simulink model "assignment2_group39_v10_final"  (R2022b)
settings: Solver=FixedStepAuto  StartTime=0.0  StopTime=30  FixedStep=0.001  RelTol=1e-3  EnableMultiTasking=on
undefined symbols (not defined in the file): A0, A1, D0, D1, D10, D11, D12, D13, D2, D3, D4, D5, D6, D7, D8, D9, PTA0, PTA1, PTA2, PTB2, PTB23, PTB3, PTB9, PTC16, PTC17, PTC2, PTC3, PTC4, PTD0, PTD1, PTD2, PTD3
libraries: frdmk64flib x24, etargetslib x16, dspstat3 x1
settings Model: ExtModeTrigDuration=5  Creator=andre  LastModifiedBy=Jack Mann
settings SolverCC: AlgebraicLoopSolver=TrustRegion
settings OptimizationCC: EnhancedBackFolding=on  PassReuseOutputArgsAs=Individual arguments  ZeroExternalMemoryAtStartup=off  ZeroInternalMemoryAtStartup=off  MaxStackSize=64  OptimizeBlockOrder=speed  DifferentSizesBufferReuse=on  OptimizationCustomize=off  EfficientTunableParamExpr=on
settings DebuggingCC: ParameterTunabilityLossMsg=error  UnconnectedInputMsg=warning  UnconnectedOutputMsg=warning  UnconnectedLineMsg=warning
settings HardwareCC: ProdBitPerPointer=32  ProdBitPerSizeT=32  ProdBitPerPtrDiffT=32  ProdLargestAtomicInteger=Long  ProdLargestAtomicFloat=Double  ProdWordSize=32  ProdHWDeviceType=ARM Compatible->ARM Cortex
settings ModelReferenceCC: EnableRefExpFcnMdlSchedulingChecks=on
settings SFSimCC: MATLABDynamicMemAlloc=off
settings RTWCC: Description=Embedded Coder  SystemTargetFile=ert.tlc  HardwareBoard=NXP FRDM-K64F  TLCOptions="-aInlineSetEventsForThisBaseRateFcn=TLC_FALSE -aSuppressMultiTaskScheduler=TLC_FALSE  -aRateBasedStepFcn=0"  TemplateMakefile=ert_default_tmf  Toolchain=GNU Tools for ARM Embedded Processors
settings CodeAppCC: ForceParamTrailComments=on  IgnoreCustomStorageClasses=off  OperatorAnnotations=on  SimulinkDataObjDesc=on  SFDataObjDesc=on  InsertBlockDesc=on

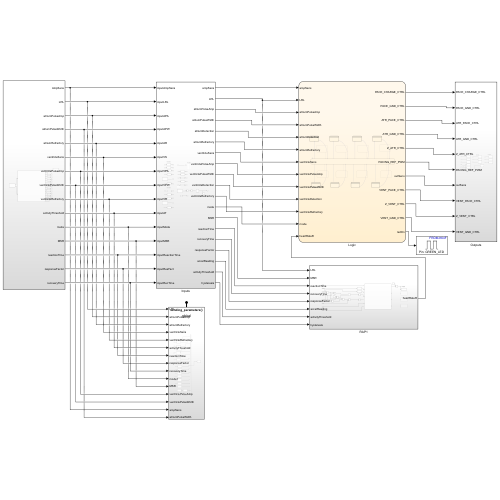
[thumbnail: Simulink's stored preview of the top-level diagram]
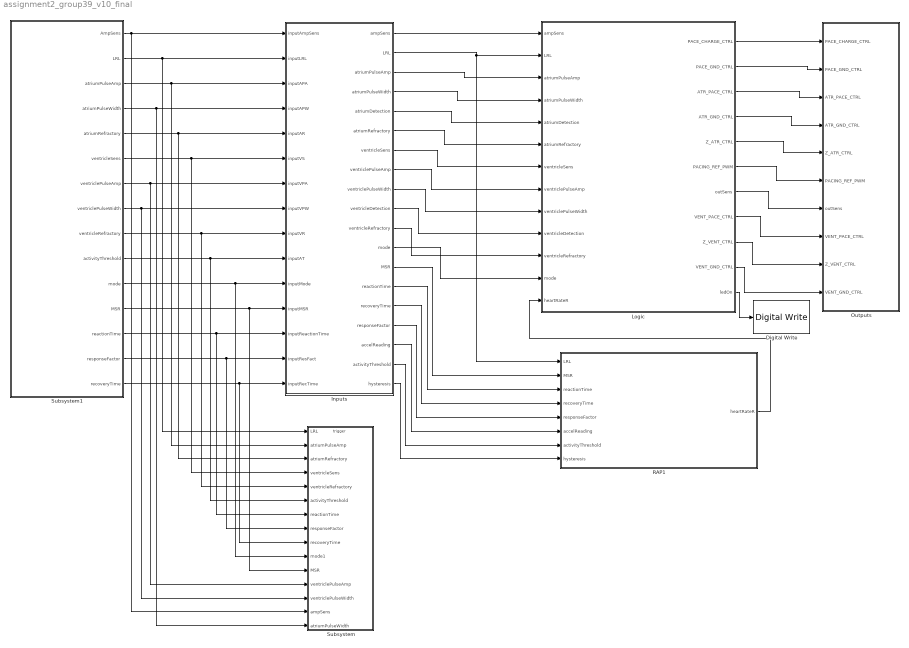
== system assignment2_group39_v10_final ==
  Digital Write : frdmk64flib/Digital Write  Whichpin=GREEN_LED
  Inputs : Subsystem
  Logic : Stateflow chart  TreatAsAtomicUnit=on
  Outputs : Subsystem
  RAP1 : Subsystem
  Subsystem : Subsystem
  Subsystem1 : Subsystem
  wires:
  Inputs/1(ampSens) -> Logic/1(ampSens)
  Inputs/2(LRL) -> RAP1/1(LRL), Logic/2(LRL)
  Inputs/3(atriumPulseAmp) -> Logic/3(atriumPulseAmp)
  Inputs/4(atriumPulseWidth) -> Logic/4(atriumPulseWidth)
  Inputs/5(atriumDetection) -> Logic/5(atriumDetection)
  Inputs/6(atriumRefractory) -> Logic/6(atriumRefractory)
  Logic/1(PACE_CHARGE_CTRL) -> Outputs/1(PACE_CHARGE_CTRL)
  Logic/2(PACE_GND_CTRL) -> Outputs/2(PACE_GND_CTRL)
  Logic/3(ATR_PACE_CTRL) -> Outputs/3(ATR_PACE_CTRL)
  Logic/4(ATR_GND_CTRL) -> Outputs/4(ATR_GND_CTRL)
  Logic/5(Z_ATR_CTRL) -> Outputs/5(Z_ATR_CTRL)
  Logic/6(PACING_REF_PWM) -> Outputs/6(PACING_REF_PWM)
  Logic/7(outSens) -> Outputs/7(outSens)
  Inputs/7(ventricleSens) -> Logic/7(ventricleSens)
  Inputs/8(ventriclePulseAmp) -> Logic/8(ventriclePulseAmp)
  Inputs/9(ventriclePulseWidth) -> Logic/9(ventriclePulseWidth)
  Inputs/10(ventricleDetection) -> Logic/10(ventricleDetection)
  Inputs/11(ventricleRefractory) -> Logic/11(ventricleRefractory)
  Logic/8(VENT_PACE_CTRL) -> Outputs/8(VENT_PACE_CTRL)
  Logic/9(Z_VENT_CTRL) -> Outputs/9(Z_VENT_CTRL)
  Logic/10(VENT_GND_CTRL) -> Outputs/10(VENT_GND_CTRL)
  Inputs/12(mode) -> Logic/12(mode)
  Inputs/13(MSR) -> RAP1/2(MSR)
  Inputs/16(responseFactor) -> RAP1/5(responseFactor)
  Inputs/14(reactionTime) -> RAP1/3(reactionTime)
  Inputs/15(recoveryTime) -> RAP1/4(recoveryTime)
  Inputs/18(activityThreshold) -> RAP1/7(activityThreshold)
  Inputs/17(accelReading) -> RAP1/6(accelReading)
  RAP1/1(heartRateR) -> Logic/13(heartRateR)
  Subsystem1/1(AmpSens) -> Subsystem/14(ampSens), Inputs/1(inputAmpSens)
  Subsystem1/3(atriumPulseAmp) -> Subsystem/2(atriumPulseAmp), Inputs/3(inputAPA)
  Subsystem1/4(atriumPulseWidth) -> Subsystem/15(atriumPulseWidth), Inputs/4(inputAPW)
  Subsystem1/6(ventricleSens) -> Subsystem/4(ventricleSens), Inputs/6(inputVS)
  Subsystem1/7(ventriclePulseAmp) -> Subsystem/12(ventriclePulseAmp), Inputs/7(inputVPA)
  Subsystem1/8(ventriclePulseWidth) -> Subsystem/13(ventriclePulseWidth), Inputs/8(inputVPW)
  Subsystem1/9(ventricleRefractory) -> Subsystem/5(ventricleRefractory), Inputs/9(inputVR)
  Subsystem1/14(responseFactor) -> Subsystem/8(responseFactor), Inputs/14(inputResFact)
  Subsystem1/15(recoveryTime) -> Subsystem/9(recoveryTime), Inputs/15(inputRecTime)
  Subsystem1/10(activityThreshold) -> Subsystem/6(activityThreshold), Inputs/10(inputAT)
  Subsystem1/11(mode) -> Subsystem/10(mode1), Inputs/11(inputMode)
  Subsystem1/12(MSR) -> Subsystem/11(MSR), Inputs/12(inputMSR)
  Subsystem1/13(reactionTime) -> Subsystem/7(reactionTime), Inputs/13(inputReactionTime)
  Inputs/19(hysteresis) -> RAP1/8(hysteresis)
  Subsystem1/2(LRL) -> Subsystem/1(LRL), Inputs/2(inputLRL)
  Subsystem1/5(atriumRefractory) -> Subsystem/3(atriumRefractory), Inputs/5(inputAR)
  Logic/11(ledOn) -> Digital Write/1

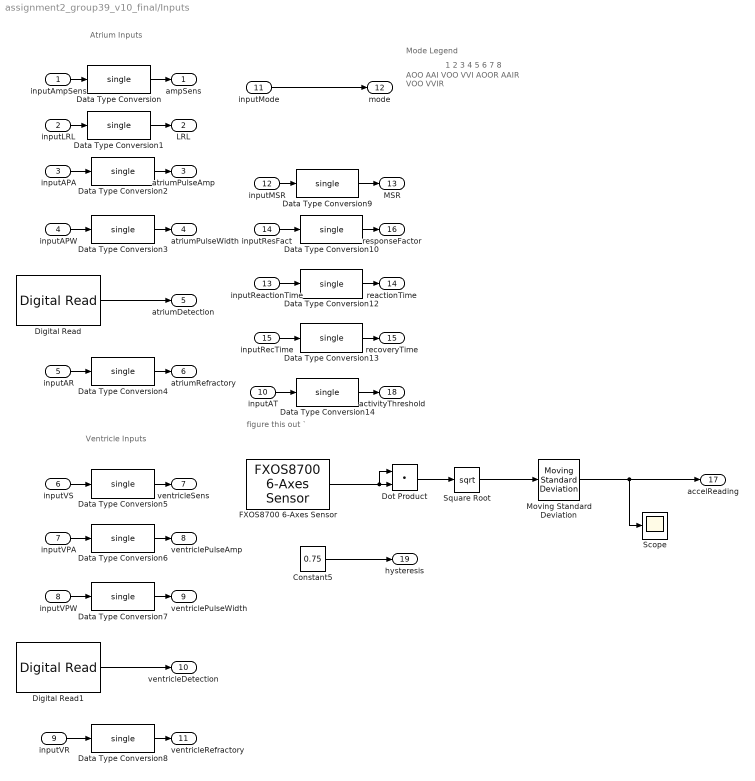
== system assignment2_group39_v10_final/Inputs ==
  note: 1
      | 2
      | 3
      | 4
      | 5
      | 6
      | 7
      | 8
  note: figure this out
      | `
  note: Mode Legend
  note: AOO
      | AAI
      | VOO
      | VVI
      | AOOR
      | AAIR
      | VOO
      | VVIR
  note: Ventricle Inputs
  note: Atrium Inputs
  inputAmpSens : Inport
  inputLRL : Inport  Port=2
  inputAPA : Inport  Port=3
  inputAPW : Inport  Port=4
  inputAR : Inport  Port=5
  inputVS : Inport  Port=6
  inputVPA : Inport  Port=7
  inputVPW : Inport  Port=8
  inputVR : Inport  Port=9
  inputAT : Inport  Port=10
  inputMode : Inport  Port=11
  inputMSR : Inport  Port=12
  inputReactionTime : Inport  Port=13
  inputResFact : Inport  Port=14
  inputRecTime : Inport  Port=15
  Constant5 : Constant  Value=0.75
  Data Type Conversion{,1..10,12..14} (14 alike) : DataTypeConversion  OutDataTypeStr=single  SaturateOnIntegerOverflow=off  RndMeth=Floor
  Digital Read : frdmk64flib/Digital Read  Whichpin=PTC16 (D0)  SampleTime=-1
  Digital Read1 : frdmk64flib/Digital Read  Whichpin=PTC17 (D1)  SampleTime=-1
  Dot Product : DotProduct  OutDataTypeStr=Inherit: Inherit via internal rule
  FXOS8700 6-Axes Sensor : frdmk64flib/FXOS8700 6-Axes Sensor  Activesensor=Accelerometer only  ODR=800Hz  HybridODR=400Hz  Accelfullrange=-4g to +4g  SampleTime=-1
  Moving Standard Deviation : dspstat3/Moving Standard Deviation  Method=Sliding window  ForgettingFactorPort=off  SpecifyWindowLength=on  WindowLength=4  OverlapLength=3  AllowArbitraryInputLength=off  ForgettingFactor=0.9  SimulateUsing=Code generation
  Scope : Scope
  Square Root : Sqrt
  ampSens : Outport  OutDataTypeStr=single
  LRL : Outport  Port=2  OutDataTypeStr=single
  atriumPulseAmp : Outport  Port=3  OutDataTypeStr=single
  atriumPulseWidth : Outport  Port=4  OutDataTypeStr=single
  atriumDetection : Outport  Port=5  OutDataTypeStr=boolean
  atriumRefractory : Outport  Port=6  OutDataTypeStr=single
  ventricleSens : Outport  Port=7  OutDataTypeStr=single
  ventriclePulseAmp : Outport  Port=8  OutDataTypeStr=single
  ventriclePulseWidth : Outport  Port=9  OutDataTypeStr=single
  ventricleDetection : Outport  Port=10  OutDataTypeStr=boolean
  ventricleRefractory : Outport  Port=11  OutDataTypeStr=single
  mode : Outport  Port=12  OutDataTypeStr=uint8
  MSR : Outport  Port=13
  reactionTime : Outport  Port=14
  recoveryTime : Outport  Port=15
  responseFactor : Outport  Port=16
  accelReading : Outport  Port=17
  activityThreshold : Outport  Port=18
  hysteresis : Outport  Port=19
  wires:
  inputAmpSens/1 -> Data Type Conversion/1
  inputAPW/1 -> Data Type Conversion3/1
  inputAR/1 -> Data Type Conversion4/1
  inputAPA/1 -> Data Type Conversion2/1
  inputLRL/1 -> Data Type Conversion1/1
  Digital Read/1 -> atriumDetection/1
  Digital Read1/1 -> ventricleDetection/1
  inputVPW/1 -> Data Type Conversion7/1
  inputVPA/1 -> Data Type Conversion6/1
  inputVR/1 -> Data Type Conversion8/1
  inputVS/1 -> Data Type Conversion5/1
  inputMSR/1 -> Data Type Conversion9/1
  inputResFact/1 -> Data Type Conversion10/1
  inputReactionTime/1 -> Data Type Conversion12/1
  inputRecTime/1 -> Data Type Conversion13/1
  inputAT/1 -> Data Type Conversion14/1
  FXOS8700 6-Axes Sensor/1 -> Dot Product/1, Dot Product/2
  Dot Product/1 -> Square Root/1
  Square Root/1 -> Moving Standard Deviation/1
  Data Type Conversion/1 -> ampSens/1
  Data Type Conversion1/1 -> LRL/1
  Data Type Conversion2/1 -> atriumPulseAmp/1
  Data Type Conversion3/1 -> atriumPulseWidth/1
  Data Type Conversion4/1 -> atriumRefractory/1
  Data Type Conversion5/1 -> ventricleSens/1
  Data Type Conversion6/1 -> ventriclePulseAmp/1
  Data Type Conversion7/1 -> ventriclePulseWidth/1
  Data Type Conversion8/1 -> ventricleRefractory/1
  Data Type Conversion9/1 -> MSR/1
  Data Type Conversion10/1 -> responseFactor/1
  inputMode/1 -> mode/1
  Data Type Conversion12/1 -> reactionTime/1
  Data Type Conversion13/1 -> recoveryTime/1
  Data Type Conversion14/1 -> activityThreshold/1
  Constant5/1 -> hysteresis/1
  Moving Standard Deviation/1 -> Scope/1, accelReading/1

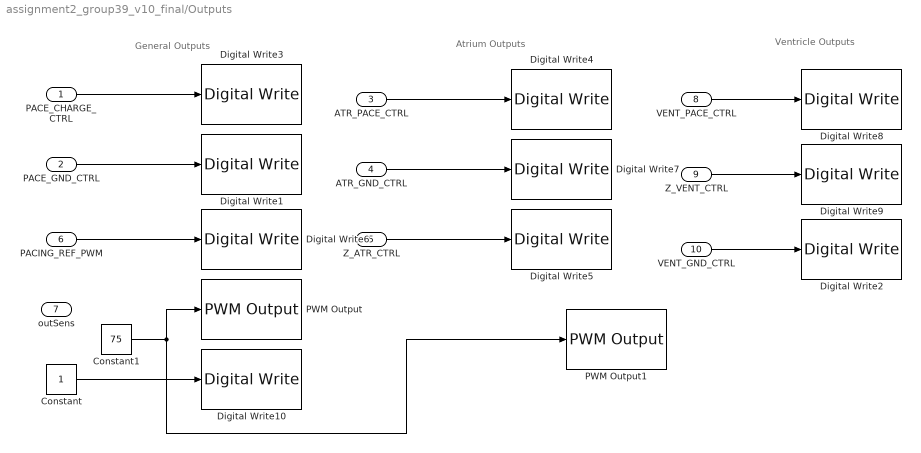
== system assignment2_group39_v10_final/Outputs ==
  note: Ventricle Outputs
  note: Atrium Outputs
  note: General Outputs
  PACE_CHARGE_CTRL : Inport  OutDataTypeStr=boolean
  PACE_GND_CTRL : Inport  Port=2  OutDataTypeStr=boolean
  ATR_PACE_CTRL : Inport  Port=3  OutDataTypeStr=boolean
  ATR_GND_CTRL : Inport  Port=4  OutDataTypeStr=boolean
  Z_ATR_CTRL : Inport  Port=5  OutDataTypeStr=boolean
  PACING_REF_PWM : Inport  Port=6  OutDataTypeStr=single
  outSens : Inport  Port=7  OutDataTypeStr=single
  VENT_PACE_CTRL : Inport  Port=8  OutDataTypeStr=boolean
  Z_VENT_CTRL : Inport  Port=9  OutDataTypeStr=boolean
  VENT_GND_CTRL : Inport  Port=10  OutDataTypeStr=boolean
  Constant : Constant  OutDataTypeStr=single
  Constant1 : Constant  Value=75
  Digital Write1 : frdmk64flib/Digital Write  Whichpin=PTD0 (D10)
  Digital Write10 : frdmk64flib/Digital Write  Whichpin=PTD1 (D13)
  Digital Write2 : frdmk64flib/Digital Write  Whichpin=PTD3 (D12)
  Digital Write3 : frdmk64flib/Digital Write  Whichpin=PTB9 (D2)
  Digital Write4 : frdmk64flib/Digital Write  Whichpin=PTA0 (D8)
  Digital Write5 : frdmk64flib/Digital Write  Whichpin=PTB23 (D4)
  Digital Write6 : frdmk64flib/Digital Write  Whichpin=PTA2 (D5)
  Digital Write7 : frdmk64flib/Digital Write  Whichpin=PTD2 (D11)
  Digital Write8 : frdmk64flib/Digital Write  Whichpin=PTC4 (D9)
  Digital Write9 : frdmk64flib/Digital Write  Whichpin=PTC3 (D7)
  PWM Output : frdmk64flib/PWM Output  Whichpin=PTC2 (D6)  InitialFrequency=2000  InitialDutyCycle=0
  PWM Output1 : frdmk64flib/PWM Output  Whichpin=PTA1 (D3)  InitialFrequency=2000  InitialDutyCycle=0
  wires:
  PACING_REF_PWM/1 -> Digital Write6/1
  ATR_PACE_CTRL/1 -> Digital Write4/1
  PACE_CHARGE_CTRL/1 -> Digital Write3/1
  Z_ATR_CTRL/1 -> Digital Write5/1
  ATR_GND_CTRL/1 -> Digital Write7/1
  Constant/1 -> Digital Write10/1
  PACE_GND_CTRL/1 -> Digital Write1/1
  Z_VENT_CTRL/1 -> Digital Write9/1
  VENT_GND_CTRL/1 -> Digital Write2/1
  VENT_PACE_CTRL/1 -> Digital Write8/1
  Constant1/1 -> PWM Output1/1, PWM Output/1

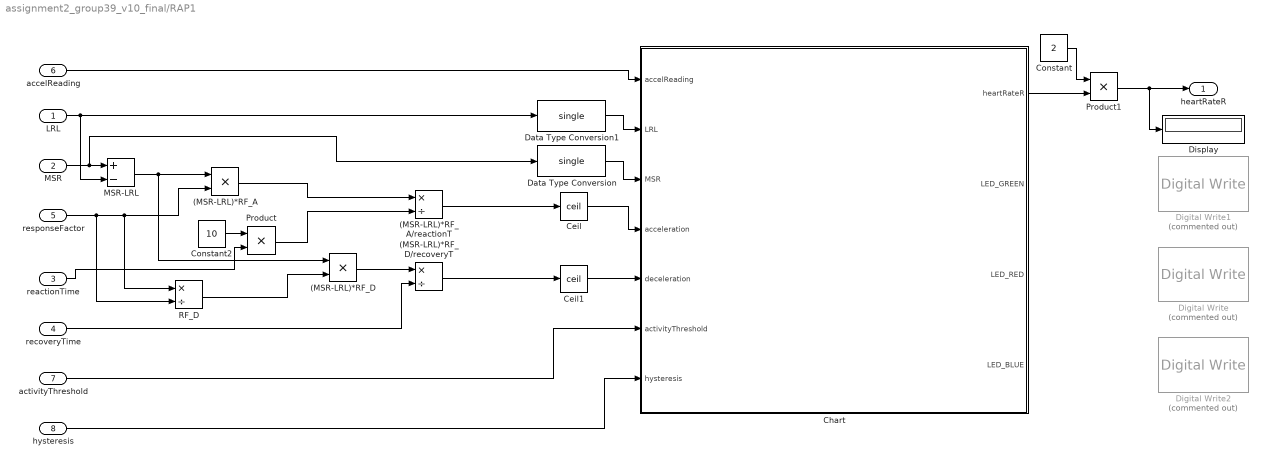
== system assignment2_group39_v10_final/RAP1 ==
  LRL : Inport
  MSR : Inport  Port=2
  reactionTime : Inport  Port=3
  recoveryTime : Inport  Port=4
  responseFactor : Inport  Port=5
  accelReading : Inport  Port=6
  activityThreshold : Inport  Port=7
  hysteresis : Inport  Port=8
  (MSR-LRL)*RF_A : Product
  (MSR-LRL)*RF_A/reactionT : Product  Inputs=*/
  (MSR-LRL)*RF_D : Product
  (MSR-LRL)*RF_D/recoveryT : Product  Inputs=*/
  Ceil : Rounding  Operator=ceil
  Ceil1 : Rounding  Operator=ceil
  Chart : Stateflow chart  TreatAsAtomicUnit=on
      settings: PortSchema="{\"entries\":[{\"content\":{\"sides\":[{\"content\":{\"connectorIds\":[\"In4\",\"In1\",\"In6\",\"In2\",\"In5\",\"In3\",\"In7\"]},\"type\":\"ConnectorPlacement.EquallySpacedRectSide\",\"uuid\":\"e727a920-989a-48c2-8c82-674329886a5f\"},{\"content\":{\"connectorIds\":[\"Out1\",\"Out3\",\"Out2\",\"Out4\"],\"side\":\"RIGHT\"},\"type\":\"ConnectorPlacement.EquallySpacedRectSide\",\"uuid\":\"1ee40f3e-9295-4daa-a641-24f0111d1364\"},{\"content\":{\"side\":\"TOP\"},\"type\":\"ConnectorPlacement.EquallySpacedRectSide\",\"uuid\":\"e3e534e8-f7ca-4b9e-96df-b8a39382b9c4\"}]},\"type\":\"ConnectorPlacement.EquallySpacedConnector\",\"uuid\":\"172b69cd-74db-4b29-a177-e1757147670c\"}],\"packageUris\":[\"http://schema.mathworks.com/mf0/Connector/R2020b\"],\"version\":\"1.0\"}"
  Constant : Constant  Value=2  OutDataTypeStr=single
  Constant2 : Constant  Value=10
  Data Type Conversion : DataTypeConversion  OutDataTypeStr=single  SaturateOnIntegerOverflow=off  RndMeth=Floor
  Data Type Conversion1 : DataTypeConversion  OutDataTypeStr=single  SaturateOnIntegerOverflow=off  RndMeth=Floor
  Digital Write : frdmk64flib/Digital Write  Commented=on  Whichpin=RED_LED
  Digital Write1 : frdmk64flib/Digital Write  Commented=on  Whichpin=GREEN_LED
  Digital Write2 : frdmk64flib/Digital Write  Commented=on  Whichpin=BLUE_LED
  Display : Display
  MSR-LRL : Sum  Inputs=+-
  Product : Product
  Product1 : Product
  RF_D : Product  Inputs=*/
  heartRateR : Outport
  wires:
  LRL/1 -> MSR-LRL/2, Data Type Conversion1/1
  accelReading/1 -> Chart/4(accelReading)
  MSR/1 -> Data Type Conversion/1, MSR-LRL/1
  MSR-LRL/1 -> (MSR-LRL)*RF_D/1, (MSR-LRL)*RF_A/1
  responseFactor/1 -> RF_D/2, RF_D/1, (MSR-LRL)*RF_A/2
  (MSR-LRL)*RF_A/1 -> (MSR-LRL)*RF_A/reactionT/1
  recoveryTime/1 -> (MSR-LRL)*RF_D/recoveryT/2
  Ceil/1 -> Chart/2(acceleration)
  (MSR-LRL)*RF_A/reactionT/1 -> Ceil/1
  (MSR-LRL)*RF_D/1 -> (MSR-LRL)*RF_D/recoveryT/1
  (MSR-LRL)*RF_D/recoveryT/1 -> Ceil1/1
  activityThreshold/1 -> Chart/3(activityThreshold)
  hysteresis/1 -> Chart/7(hysteresis)
  Data Type Conversion/1 -> Chart/6(MSR)
  Data Type Conversion1/1 -> Chart/1(LRL)
  Product1/1 -> heartRateR/1, Display/1
  Ceil1/1 -> Chart/5(deceleration)
  Product/1 -> (MSR-LRL)*RF_A/reactionT/2
  Constant2/1 -> Product/1
  reactionTime/1 -> Product/2
  RF_D/1 -> (MSR-LRL)*RF_D/2
  Chart/1(heartRateR) -> Product1/2
  Constant/1 -> Product1/1

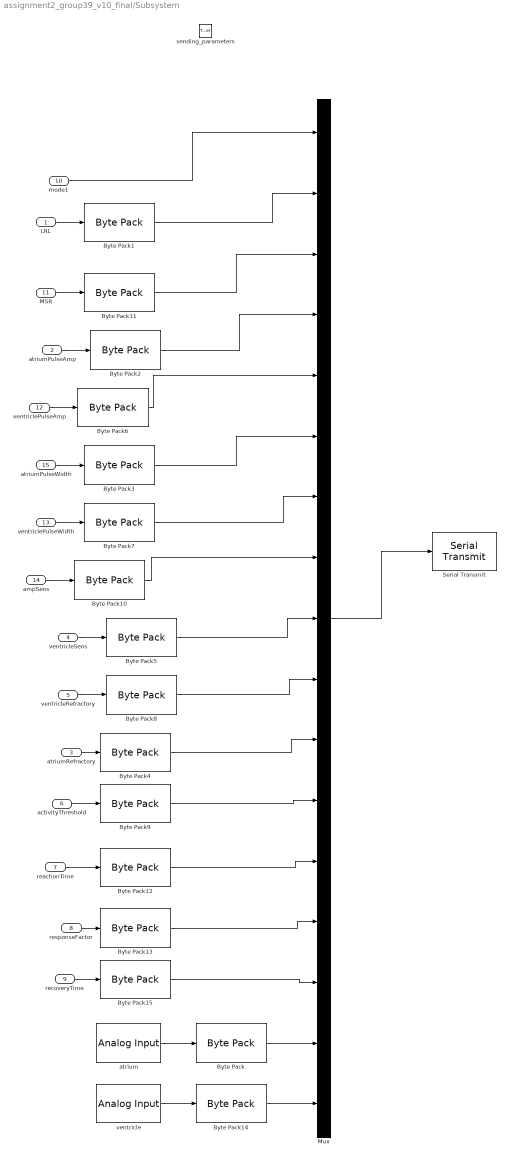
== system assignment2_group39_v10_final/Subsystem ==
  LRL : Inport  OutDataTypeStr=double
  atriumPulseAmp : Inport  Port=2  OutDataTypeStr=double
  atriumRefractory : Inport  Port=3  OutDataTypeStr=double
  ventricleSens : Inport  Port=4  OutDataTypeStr=double
  ventricleRefractory : Inport  Port=5  OutDataTypeStr=double
  activityThreshold : Inport  Port=6  OutDataTypeStr=double
  reactionTime : Inport  Port=7  OutDataTypeStr=double
  responseFactor : Inport  Port=8  OutDataTypeStr=double
  recoveryTime : Inport  Port=9  OutDataTypeStr=double
  mode1 : Inport  Port=10  OutDataTypeStr=uint8
  MSR : Inport  Port=11  OutDataTypeStr=double
  ventriclePulseAmp : Inport  Port=12  OutDataTypeStr=double
  ventriclePulseWidth : Inport  Port=13  OutDataTypeStr=double
  ampSens : Inport  Port=14  OutDataTypeStr=double
  atriumPulseWidth : Inport  Port=15  OutDataTypeStr=double
  sending_parameters : TriggerPort  TriggerType=function-call  IsSimulinkFunction=on  FunctionName=sending_parameters  VariantControl=Variant
  Byte Pack{,1..15} (16 alike) : etargetslib/Byte Pack  datatypes={'double'}  byteAlign=1
  Mux : Mux  Inputs=17
  Serial Transmit : frdmk64flib/Serial Transmit  SCIModule=0  Baudrate=uint32(9600)  Parity=None  StopBits=1  HardwareFlowControl=None  ByteOrder=LittleEndian  BlockingMode=on  OutputStatus=off
  atrium : frdmk64flib/Analog Input  Whichpin=PTB2 (A0)  SampleTime=-1
  ventricle : frdmk64flib/Analog Input  Whichpin=PTB3 (A1)  SampleTime=-1
  wires:
  LRL/1 -> Byte Pack1/1
  atriumPulseAmp/1 -> Byte Pack2/1
  atriumRefractory/1 -> Byte Pack4/1
  ventricleSens/1 -> Byte Pack5/1
  ventricleRefractory/1 -> Byte Pack8/1
  activityThreshold/1 -> Byte Pack9/1
  reactionTime/1 -> Byte Pack12/1
  responseFactor/1 -> Byte Pack13/1
  recoveryTime/1 -> Byte Pack15/1
  Mux/1 -> Serial Transmit/1
  MSR/1 -> Byte Pack11/1
  Byte Pack11/1 -> Mux/3
  ventriclePulseAmp/1 -> Byte Pack6/1
  ventriclePulseWidth/1 -> Byte Pack7/1
  ampSens/1 -> Byte Pack10/1
  atriumPulseWidth/1 -> Byte Pack3/1
  Byte Pack15/1 -> Mux/15
  Byte Pack13/1 -> Mux/14
  Byte Pack12/1 -> Mux/13
  Byte Pack9/1 -> Mux/12
  Byte Pack4/1 -> Mux/11
  Byte Pack8/1 -> Mux/10
  Byte Pack5/1 -> Mux/9
  Byte Pack10/1 -> Mux/8
  Byte Pack7/1 -> Mux/7
  Byte Pack3/1 -> Mux/6
  Byte Pack6/1 -> Mux/5
  Byte Pack2/1 -> Mux/4
  Byte Pack1/1 -> Mux/2
  mode1/1 -> Mux/1
  atrium/1 -> Byte Pack/1
  ventricle/1 -> Byte Pack14/1
  Byte Pack/1 -> Mux/16
  Byte Pack14/1 -> Mux/17

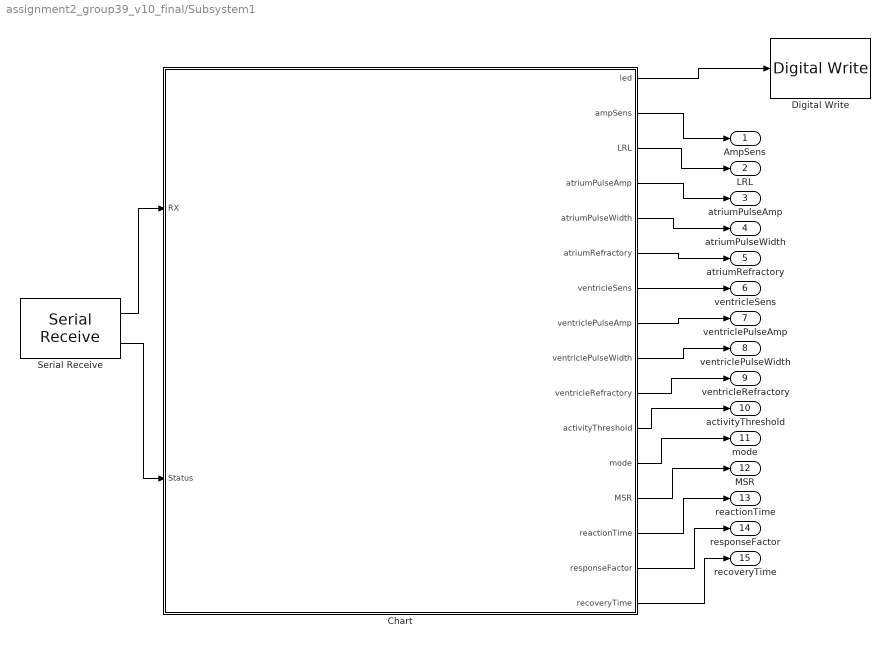
== system assignment2_group39_v10_final/Subsystem1 ==
  Chart : Stateflow chart  TreatAsAtomicUnit=on
      settings: PortSchema="{\"entries\":[{\"content\":{\"sides\":[{\"content\":{\"connectorIds\":[\"In2\",\"In1\"]},\"type\":\"ConnectorPlacement.EquallySpacedRectSide\",\"uuid\":\"4f5a3770-f300-418f-9487-637399e38c69\"},{\"content\":{\"connectorIds\":[\"Out1\",\"Out2\",\"Out3\",\"Out4\",\"Out5\",\"Out6\",\"Out7\",\"Out8\",\"Out9\",\"Out16\",\"Out10\",\"Out11\",\"Out12\",\"Out13\",\"Out14\",\"Out15\"],\"side\":\"RIGHT\"},\"type\":\"ConnectorPlacement.EquallySpacedRectSide\",\"uuid\":\"cfe58ccd-6f5b-444c-9e2a-780fa37746c4\"},{\"content\":{\"side\":\"TOP\"},\"type\":\"ConnectorPlacement.EquallySpacedRectSide\",\"uuid\":\"1127273a-22ba-4ea7-9f5a-6224bf23e303\"}]},\"type\":\"ConnectorPlacement.EquallySpacedConnector\",\"uuid\":\"786a0154-0823-4f04-a45d-1bc6ecdd10fe\"}],\"packageUris\":[\"http://schema.mathworks.com/mf0/Connector/R2020b\"],\"version\":\"1.0\"}"
  Digital Write : frdmk64flib/Digital Write  Whichpin=BLUE_LED
  Serial Receive : frdmk64flib/Serial Receive  SCIModule=0  Baudrate=uint32(9600)  Parity=None  StopBits=1  HardwareFlowControl=None  ByteOrder=LittleEndian  DataType=uint8  DataLength=115  BlockingMode=off  OutputStatus=on  SampleTime=0.1
  AmpSens : Outport  OutDataTypeStr=double
  LRL : Outport  Port=2  OutDataTypeStr=double
  atriumPulseAmp : Outport  Port=3  OutDataTypeStr=double
  atriumPulseWidth : Outport  Port=4  OutDataTypeStr=double
  atriumRefractory : Outport  Port=5  OutDataTypeStr=double
  ventricleSens : Outport  Port=6  OutDataTypeStr=double
  ventriclePulseAmp : Outport  Port=7  OutDataTypeStr=double
  ventriclePulseWidth : Outport  Port=8  OutDataTypeStr=double
  ventricleRefractory : Outport  Port=9  OutDataTypeStr=double
  activityThreshold : Outport  Port=10  OutDataTypeStr=double
  mode : Outport  Port=11  OutDataTypeStr=uint8
  MSR : Outport  Port=12  OutDataTypeStr=double
  reactionTime : Outport  Port=13  OutDataTypeStr=double
  responseFactor : Outport  Port=14  OutDataTypeStr=double
  recoveryTime : Outport  Port=15  OutDataTypeStr=double
  wires:
  Serial Receive/1 -> Chart/2(RX)
  Serial Receive/2 -> Chart/1(Status)
  Chart/1(led) -> Digital Write/1
  Chart/2(ampSens) -> AmpSens/1
  Chart/3(LRL) -> LRL/1
  Chart/4(atriumPulseAmp) -> atriumPulseAmp/1
  Chart/5(atriumPulseWidth) -> atriumPulseWidth/1
  Chart/6(atriumRefractory) -> atriumRefractory/1
  Chart/7(ventricleSens) -> ventricleSens/1
  Chart/8(ventriclePulseAmp) -> ventriclePulseAmp/1
  Chart/9(ventriclePulseWidth) -> ventriclePulseWidth/1
  Chart/10(activityThreshold) -> activityThreshold/1
  Chart/11(mode) -> mode/1
  Chart/12(MSR) -> MSR/1
  Chart/13(reactionTime) -> reactionTime/1
  Chart/14(responseFactor) -> responseFactor/1
  Chart/15(recoveryTime) -> recoveryTime/1
  Chart/16(ventricleRefractory) -> ventricleRefractory/1

== stateflow chart assignment2_group39_v10_final/Subsystem1/Chart ==
  state ECHO_PARAM
    entry:
    led = 0
    sending_parameters();
  state Initial
    %Setting initial values of parameters
    entry:
    ampSens = 75
    LRL = 60
    atriumPulseAmp = 3.75
    atriumPulseWidth = 0.4
    atriumRefractory = 250
    ventricleSens = 75
    ventriclePulseAmp = 3.75
    ventriclePulseWidth = 0.4
    ventricleRefractory = 250
    activityThreshold = 1
    mode = 1
    MSR = 175
    reactionTime = 0.5
    responseFactor = 8
    recoveryTime = 5
  state ParameterSet
    entry:
    led = 1
    mode = RX(3);
    LRL = typecast(RX(4:11),'double');
    MSR = typecast(RX(12:19),'double');
    atriumPulseAmp = typecast(RX(20:27),'double');
    ventriclePulseAmp = typecast(RX(28:35),'double');
    atriumPulseWidth = typecast(RX(36:43),'double');
    ventriclePulseWidth = typecast(RX(44:51),'double');
    ampSens = typecast(RX(52:59),'double');
    ventricleSens = typecast(RX(60:67),'double');
    ventricleRefractory = typecast(RX(68:75),'double');
    atriumRefractory = typecast(RX(76:83),'double');
    activityThreshold = typecast(RX(84:91),'double');
    reactionTime = typecast(RX(92:99),'double');
    responseFactor = typecast(RX(100:107),'double');
    recoveryTime = typecast(RX(108:115),'double');
  state Standby
    %Waiting for COM
  state SendBack
    entry:
    sending_parameters();
  (junction 44) -> ECHO_PARAM [order 2] : [(RX(2)) == hex2dec('02')]
  (junction 44) -> ParameterSet [order 1] : [RX(2) == hex2dec('01')]
  (junction 43) -> (junction 44) [order 1] : [(RX(1)) == hex2dec('01')]
  ECHO_PARAM -> Standby : after(1000,msec)
  (default) -> Initial
  Standby -> (junction 43) : [Status==0]
  (junction 43) -> Standby [order 2]
  Initial -> Standby
  SendBack -> Standby : after(1000,msec)
  ParameterSet -> SendBack : after(1000,msec)
  data: led output uint8; ampSens output double; LRL output double; atriumPulseAmp output double; atriumPulseWidth output double; atriumRefractory output double; ventricleSens output double; ventriclePulseAmp output double; ventriclePulseWidth output double; activityThreshold output double; mode output uint8; MSR output double; reactionTime output double; responseFactor output double; recoveryTime output double; Status input uint8; ventricleRefractory output double; RX input uint8

== stateflow chart assignment2_group39_v10_final/Logic ==
  state AOO
    state Charging_C22_Discharging_C21
      entry:
      PACING_REF_PWM=(atriumPulseAmp);
      PACE_GND_CTRL = true;
      Z_ATR_CTRL = false;
      ATR_PACE_CTRL = false;
      ATR_GND_CTRL = true;
      PACE_CHARGE_CTRL = true;
      outSens = ampSens;
      %charging primary capacitor and discharging blocking
      %capacitor in the same state
    state Pacing
      entry:
      PACE_CHARGE_CTRL = false;
      PACE_GND_CTRL = true;
      Z_ATR_CTRL = false;
      ATR_GND_CTRL = false;
      ATR_PACE_CTRL = true;
      %discharging primary capacitor for pulse width
    (default) -> AOO.Charging_C22_Discharging_C21
    AOO.Charging_C22_Discharging_C21 -> AOO.Pacing [order 1] : [after(60000/LRL-atriumPulseWidth,msec)]
    AOO.Pacing -> AOO.Charging_C22_Discharging_C21 : [after(atriumPulseWidth,msec)]
  state AAI
    state Charging_C22_Discharging_C21
      entry:
      PACING_REF_PWM=(atriumPulseAmp);
      PACE_GND_CTRL = true;
      Z_ATR_CTRL = false;
      ATR_PACE_CTRL = false;
      ATR_GND_CTRL = true;
      PACE_CHARGE_CTRL = true;
      outSens = ampSens;
      %charging primary capacitor and discharging blocking
      %capacitor in the same state
    state Pacing
      entry:
      PACE_CHARGE_CTRL = false;
      PACE_GND_CTRL = true;
      Z_ATR_CTRL = false;
      ATR_GND_CTRL = false;
      ATR_PACE_CTRL = true;
      %discharging primary capacitor for pulse width
    state Sensing
    AAI.Sensing -> AAI.Charging_C22_Discharging_C21 [order 1] : [atriumDetection==1]
    (default) -> AAI.Charging_C22_Discharging_C21
    AAI.Charging_C22_Discharging_C21 -> AAI.Sensing [order 1] : [after(atriumRefractory,msec)]
    AAI.Sensing -> AAI.Pacing [order 2] : after(60000/LRL-atriumRefractory-atriumPulseWidth,msec)[atriumDetection==0]
    AAI.Pacing -> AAI.Charging_C22_Discharging_C21 : [after(atriumPulseWidth,msec)]
  state VOO
    state Charging_C22_Discharging_C21
      entry:
      PACING_REF_PWM=(ventriclePulseAmp);
      PACE_GND_CTRL = true;
      VENT_PACE_CTRL = false;
      Z_VENT_CTRL = false;
      VENT_GND_CTRL = true;
      PACE_CHARGE_CTRL = true;
      outSens = ventricleSens;
      %charging primary capacitor and discharging blocking
      %capacitor in the same state
    state Pacing
      entry:
      PACE_CHARGE_CTRL = false;
      PACE_GND_CTRL = true;
      Z_VENT_CTRL = false;
      VENT_GND_CTRL = false;
      VENT_PACE_CTRL = true;
      %discharging primary capacitor for pulse width
    (default) -> VOO.Charging_C22_Discharging_C21
    VOO.Charging_C22_Discharging_C21 -> VOO.Pacing [order 1] : [after(60000/LRL-ventriclePulseWidth,msec)]
    VOO.Pacing -> VOO.Charging_C22_Discharging_C21 : [after(ventriclePulseWidth,msec)]
  state VVI
    state Charging_C22_Discharging_C21
      entry:
      PACING_REF_PWM=(ventriclePulseAmp);
      PACE_GND_CTRL = true;
      VENT_PACE_CTRL = false;
      Z_VENT_CTRL = false;
      VENT_GND_CTRL = true;
      PACE_CHARGE_CTRL = true;
      outSens = ventricleSens;
      period = 60000/LRL
      %charging primary capacitor and discharging blocking
      %capacitor in the same state
    state Pacing
      entry:
      PACE_CHARGE_CTRL = false;
      PACE_GND_CTRL = true;
      Z_VENT_CTRL = false;
      VENT_GND_CTRL = false;
      VENT_PACE_CTRL = true;
      ledOn = 1
      %discharging primary capacitor for pulse width
    state Sensing
    VVI.Sensing -> VVI.Charging_C22_Discharging_C21 [order 1] : [ventricleDetection==1]
    (default) -> VVI.Charging_C22_Discharging_C21
    VVI.Charging_C22_Discharging_C21 -> VVI.Sensing [order 1] : [after(ventricleRefractory,msec)]
    VVI.Sensing -> VVI.Pacing [order 2] : after(period-ventricleRefractory-ventriclePulseWidth,msec)[ventricleDetection==0]
    VVI.Pacing -> VVI.Charging_C22_Discharging_C21 : [after(ventriclePulseWidth,msec)]
  state Exit_VVI [commented out]
    entry:
    PACE_CHARGE_CTRL = false;
    PACE_GND_CTRL = true;
    Z_VENT_CTRL = false;
    VENT_GND_CTRL = false;
    VENT_PACE_CTRL = true;
  state Exit_AOO [commented out]
    entry:
    PACE_CHARGE_CTRL = false;
    PACE_GND_CTRL = true;
    Z_ATR_CTRL = false;
    ATR_GND_CTRL = false;
    ATR_PACE_CTRL = true;
  state Exit_AAI [commented out]
    entry:
    PACE_CHARGE_CTRL = false;
    PACE_GND_CTRL = true;
    Z_ATR_CTRL = false;
    ATR_GND_CTRL = false;
    ATR_PACE_CTRL = true;
  state Exit_VOO [commented out]
    entry:
    PACE_CHARGE_CTRL = false;
    PACE_GND_CTRL = true;
    Z_VENT_CTRL = false;
    VENT_GND_CTRL = false;
    VENT_PACE_CTRL = true;
  state Default
  state Exit_AOOR [commented out]
    entry:
    PACE_CHARGE_CTRL = false;
    PACE_GND_CTRL = true;
    Z_ATR_CTRL = false;
    ATR_GND_CTRL = false;
    ATR_PACE_CTRL = true;
  state Exit_AAIR [commented out]
    entry:
    PACE_CHARGE_CTRL = false;
    PACE_GND_CTRL = true;
    Z_ATR_CTRL = false;
    ATR_GND_CTRL = false;
    ATR_PACE_CTRL = true;
  state Exit_VOOR [commented out]
    entry:
    PACE_CHARGE_CTRL = false;
    PACE_GND_CTRL = true;
    Z_VENT_CTRL = false;
    VENT_GND_CTRL = false;
    VENT_PACE_CTRL = true;
  state Exit_VVIR [commented out]
    entry:
    PACE_CHARGE_CTRL = false;
    PACE_GND_CTRL = true;
    Z_VENT_CTRL = false;
    VENT_GND_CTRL = false;
    VENT_PACE_CTRL = true;
  state VOOR
    state Charging_C22_Discharging_C21
      entry:
      PACING_REF_PWM=(ventriclePulseAmp);
      PACE_GND_CTRL = true;
      VENT_PACE_CTRL = false;
      Z_VENT_CTRL = false;
      VENT_GND_CTRL = true;
      PACE_CHARGE_CTRL = true;
      outSens = ventricleSens;
      %charging primary capacitor and discharging blocking
      %capacitor in the same state
    state Pacing
      entry:
      PACE_CHARGE_CTRL = false;
      PACE_GND_CTRL = true;
      Z_VENT_CTRL = false;
      VENT_GND_CTRL = false;
      VENT_PACE_CTRL = true;
      %discharging primary capacitor for pulse width
    (default) -> VOOR.Charging_C22_Discharging_C21
    VOOR.Charging_C22_Discharging_C21 -> VOOR.Pacing [order 2] : [after(60000/heartRateR-ventriclePulseWidth,msec)]
    VOOR.Pacing -> VOOR.Charging_C22_Discharging_C21 : [after(ventriclePulseWidth,msec)]
  state VVIR
    state Charging_C22_Discharging_C21
      entry:
      PACING_REF_PWM=(ventriclePulseAmp);
      PACE_GND_CTRL = true;
      VENT_PACE_CTRL = false;
      Z_VENT_CTRL = false;
      VENT_GND_CTRL = true;
      PACE_CHARGE_CTRL = true;
      outSens = ventricleSens;
      %charging primary capacitor and discharging blocking
      %capacitor in the same state
    state Pacing
      entry:
      PACE_CHARGE_CTRL = false;
      PACE_GND_CTRL = true;
      Z_VENT_CTRL = false;
      VENT_GND_CTRL = false;
      VENT_PACE_CTRL = true;
      %discharging primary capacitor for pulse width
    state Sensing
    VVIR.Sensing -> VVIR.Charging_C22_Discharging_C21 [order 1] : [ventricleDetection==1]
    (default) -> VVIR.Charging_C22_Discharging_C21
    VVIR.Charging_C22_Discharging_C21 -> VVIR.Sensing [order 1] : [after(ventricleRefractory,msec)]
    VVIR.Sensing -> VVIR.Pacing [order 2] : after(60000/heartRateR-ventricleRefractory-ventriclePulseWidth,msec)[ventricleDetection==0]
    VVIR.Pacing -> VVIR.Charging_C22_Discharging_C21 : [after(ventriclePulseWidth,msec)]
  state AOOR
    state Charging_C22_Discharging_C21
      entry:
      PACING_REF_PWM=(atriumPulseAmp);
      PACE_GND_CTRL = true;
      Z_ATR_CTRL = false;
      ATR_PACE_CTRL = false;
      ATR_GND_CTRL = true;
      PACE_CHARGE_CTRL = true;
      outSens = ampSens;
      %charging primary capacitor and discharging blocking
      %capacitor in the same state
    state Pacing
      entry:
      PACE_CHARGE_CTRL = false;
      PACE_GND_CTRL = true;
      Z_ATR_CTRL = false;
      ATR_GND_CTRL = false;
      ATR_PACE_CTRL = true;
      %discharging primary capacitor for pulse width
    (default) -> AOOR.Charging_C22_Discharging_C21
    AOOR.Charging_C22_Discharging_C21 -> AOOR.Pacing [order 2] : [after(60000/heartRateR - atriumPulseWidth,msec)]
    AOOR.Pacing -> AOOR.Charging_C22_Discharging_C21 : [after(atriumPulseWidth,msec)]
  state AAIR
    state Charging_C22_Discharging_C21
      entry:
      PACING_REF_PWM=(atriumPulseAmp);
      PACE_GND_CTRL = true;
      Z_ATR_CTRL = false;
      ATR_PACE_CTRL = false;
      ATR_GND_CTRL = true;
      PACE_CHARGE_CTRL = true;
      outSens = ampSens;
      %charging primary capacitor and discharging blocking
      %capacitor in the same state
    state Pacing
      entry:
      PACE_CHARGE_CTRL = false;
      PACE_GND_CTRL = true;
      Z_ATR_CTRL = false;
      ATR_GND_CTRL = false;
      ATR_PACE_CTRL = true;
      %discharging primary capacitor for pulse width
    state Sensing
    AAIR.Sensing -> AAIR.Charging_C22_Discharging_C21 [order 1] : [atriumDetection==1]
    (default) -> AAIR.Charging_C22_Discharging_C21
    AAIR.Charging_C22_Discharging_C21 -> AAIR.Sensing [order 1] : [after(atriumRefractory,msec)]
    AAIR.Sensing -> AAIR.Pacing [order 2] : after(60000/heartRateR-atriumRefractory-atriumPulseWidth,msec)[atriumDetection==0]
    AAIR.Pacing -> AAIR.Charging_C22_Discharging_C21 : [after(atriumPulseWidth,msec)]
  Default -> AOO [order 1] : [mode == 1]
  Default -> AAI [order 3] : [mode == 3]
  Default -> VOO [order 2] : [mode == 2]
  Default -> VVI [order 4] : [mode == 4]
  AOO.Charging_C22_Discharging_C21 -> Default [order 2] : [mode ~=1]
  VVIR.Charging_C22_Discharging_C21 -> Default [order 2] : [mode ~=8]
  AOOR.Charging_C22_Discharging_C21 -> Default [order 1] : [mode ~=5]
  VVI.Charging_C22_Discharging_C21 -> Default [order 2] : [mode ~=4]
  AAIR.Charging_C22_Discharging_C21 -> Default [order 2] : [mode ~=7]
  VOOR.Charging_C22_Discharging_C21 -> Default [order 1] : [mode ~=6]
  VOO.Charging_C22_Discharging_C21 -> Default [order 2] : [mode ~=2]
  AAI.Charging_C22_Discharging_C21 -> Default [order 2] : [mode ~=3]
  Exit_VVI -> Default [commented out]
  Exit_AOO -> Default [commented out]
  Exit_AAI -> Default [commented out]
  Exit_VOO -> Default [commented out]
  (default) -> Default
  Default -> AOOR [order 5] : [mode == 5]
  Exit_AOOR -> Default [commented out]
  Default -> AAIR [order 7] : [mode == 7]
  Exit_AAIR -> Default [commented out]
  Default -> VOOR [order 6] : [mode == 6]
  Exit_VOOR -> Default [commented out]
  Default -> VVIR [order 8] : [mode == 8]
  Exit_VVIR -> Default [commented out]
  data: ampSens input single; LRL input single; atriumPulseAmp input single; atriumPulseWidth input single; atriumDetection input boolean; atriumRefractory input single; PACE_CHARGE_CTRL output boolean; PACE_GND_CTRL output boolean; ATR_PACE_CTRL output boolean; ATR_GND_CTRL output boolean; Z_ATR_CTRL output boolean; PACING_REF_PWM output single; outSens output single; ventricleSens input single; ventriclePulseAmp input single; ventriclePulseWidth input single; ventricleDetection input boolean; ventricleRefractory input single; VENT_PACE_CTRL output boolean; Z_VENT_CTRL output boolean; VENT_GND_CTRL output boolean; mode input uint8; heartRateR input single; ledOn output; period local

== stateflow chart assignment2_group39_v10_final/RAP1/Chart ==
  note: .
  state Start_State
    entry:
    heartRateR = LRL
    LED_GREEN = false;
    LED_RED = false;
    LED_BLUE = true;
  state Acceleration_State
    entry:
    heartRateR = heartRateR + acceleration
    LED_GREEN = true;
    LED_RED = false;
    LED_BLUE = false;
  state Deceleration_State
    entry:
    heartRateR = heartRateR - deceleration
    LED_GREEN = false;
    LED_RED = true;
    LED_BLUE = false;
  state Steady_State
    entry:
    heartRateR = MSR;
    LED_GREEN = false;
    LED_RED = false;
    LED_BLUE = true;
  note: .
  (default) -> Start_State
  Start_State -> Acceleration_State : [accelReading >= activityThreshold]
  Deceleration_State -> Start_State [order 2] : [heartRateR <= LRL]
  Acceleration_State -> Acceleration_State [order 3] : after(1000, msec)[MSR > heartRateR && accelReading >= hysteresis]
  Deceleration_State -> Deceleration_State [order 3] : after(1000, msec)[heartRateR >= LRL && accelReading < hysteresis]
  Acceleration_State -> Deceleration_State [order 2] : [accelReading < hysteresis]
  Deceleration_State -> Acceleration_State [order 1] : [accelReading >= hysteresis]
  Acceleration_State -> Steady_State [order 1] : [heartRateR >= MSR]
  Steady_State -> Deceleration_State [order 1] : [accelReading < hysteresis]
  Steady_State -> Steady_State [order 2] : after(1000, msec)[accelReading > hysteresis]
  data: heartRateR output; LRL input; acceleration input; activityThreshold input; accelReading input; deceleration input; LED_RED output; LED_GREEN output; LED_BLUE output; MSR input; hysteresis input
